simulink model "PV_PEM_direct_battery_active"  (R2026a)
settings: Solver=VariableStepAuto  StopTime=sim_t
values from neighbouring files (symbols this model uses):
  Bi_L = 4e-4    (= 0.0004)    [PV_PEM_direct_battery_active.m]    (also in PV_PEM_direct_battery_passive.m; PV_PEM_indirect_battery.m; PV_PEM_reconfigurable_battery.m)
  Irr_stair_time = (0:Irr_stair_tsamp:sim_t)'    [PV_PEM_direct_battery_active.m]    (also in PV_PEM_direct_battery_passive.m = 0:Irr_stair_tsamp:sim_t; PV_PEM_indirect_battery.m; PV_PEM_reconfigurable_battery.m = (0 : Irr_stair_tsamp : sim_t)')
  Irr_stair_val = interp1(Irr_time, Irr_val, Irr_stair_time, 'linear', 0)    [PV_PEM_direct_battery_active.m]    (also in PV_PEM_direct_battery_passive.m; PV_PEM_indirect_battery.m; PV_PEM_reconfigurable_battery.m = interp1(Irr_time, Irr_val,  Irr_stair_time, 'linear', 0))
  Q_batt = 0.1    [PV_PEM_direct_battery_active.m]    (also in PV_PEM_direct_battery_passive.m; PV_PEM_indirect_battery.m; PV_PEM_reconfigurable_battery.m = 0.00694444444444)
  Ra_stack = Ra   * N    (= 0.02301)    [PV_PEM_direct_battery_active.m]    (also in PV_PEM_direct_battery_passive.m; PV_PEM_indirect_battery.m = 0.0177; PV_PEM_reconfigurable_battery.m = 0.02832)
  Rc_stack = Rc   * N    (= 0.0065)    [PV_PEM_direct_battery_active.m]    (also in PV_PEM_direct_battery_passive.m; PV_PEM_indirect_battery.m = 0.005; PV_PEM_reconfigurable_battery.m = 0.008)
  Rint_stack = Rint * N    (= 0.112749)    [PV_PEM_direct_battery_active.m]    (also in PV_PEM_direct_battery_passive.m; PV_PEM_indirect_battery.m = 0.08673; PV_PEM_reconfigurable_battery.m = 0.138768)
  sample_output_time = 1e-3    (= 0.001)    [PV_PEM_direct_battery_active.m]    (also in PV_PEM_direct_battery_passive.m = 0.0001; PV_PEM_indirect_battery.m = 0.01; PV_PEM_reconfigurable_battery.m = 0.00166666666667)
  SOC_max = 0.9    [PV_PEM_direct_battery_active.m]    (also in PV_PEM_direct_battery_passive.m = 90; PV_PEM_indirect_battery.m; PV_PEM_reconfigurable_battery.m = 90)
  SOC_min = 0.2    [PV_PEM_direct_battery_active.m]    (also in PV_PEM_direct_battery_passive.m = 20; PV_PEM_indirect_battery.m; PV_PEM_reconfigurable_battery.m = 20)
  Ts = 1e-4    (= 0.0001)    [PV_PEM_direct_battery_active.m]    (also in PV_PEM_direct_battery_passive.m; PV_PEM_indirect_battery.m = 0.001; PV_PEM_reconfigurable_battery.m)
  V_ref_battery = (Vint_stack + Vmax_PEM) / 2.1    (= 21.5171109524)    [PV_PEM_direct_battery_active.m]    (also in PV_PEM_direct_battery_passive.m = 22.5929665; PV_PEM_indirect_battery.m = 17.379205; PV_PEM_reconfigurable_battery.m = 27.806728)
libraries: fl_lib x18, nesl_utility x13, simulink x4, ee_lib x3, batteryecm_lib x1, slpidlib x1
settings Model: Creator=hanna  LastModifiedBy=Diamantis
settings SimscapeCC: SimscapeNominalValues="[{\"value\":\"1\",\"unit\":\"A\"},{\"value\":\"1\",\"unit\":\"bar\"},{\"value\":\"1\",\"unit\":\"cm^2\"},{\"value\":\"1\",\"unit\":\"cm^3/s\"},{\"value\":\"1\",\"unit\":\"kJ/kg\"},{\"value\":\"1\",\"unit\":\"kW\"},{\"value\":\"1\",\"unit\":\"l\"},{\"value\":\"1\",\"unit\":\"N\"},{\"value\":\"1\",\"unit\":\"N*m\"},{\"value\":\"1\",\"unit\":\"V\"}]"  SimscapeLogType=none  SimscapeLogDataHistory=5000.0

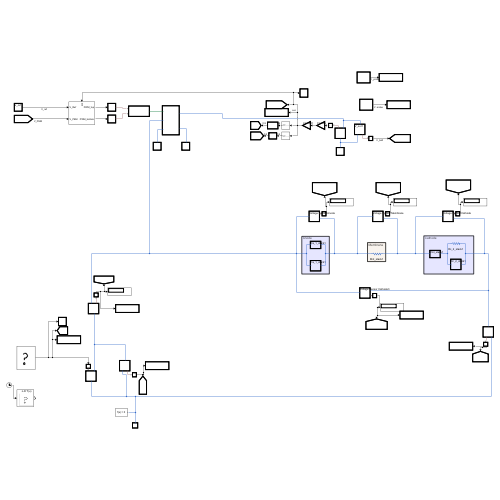
[thumbnail: Simulink's stored preview of the top-level diagram]
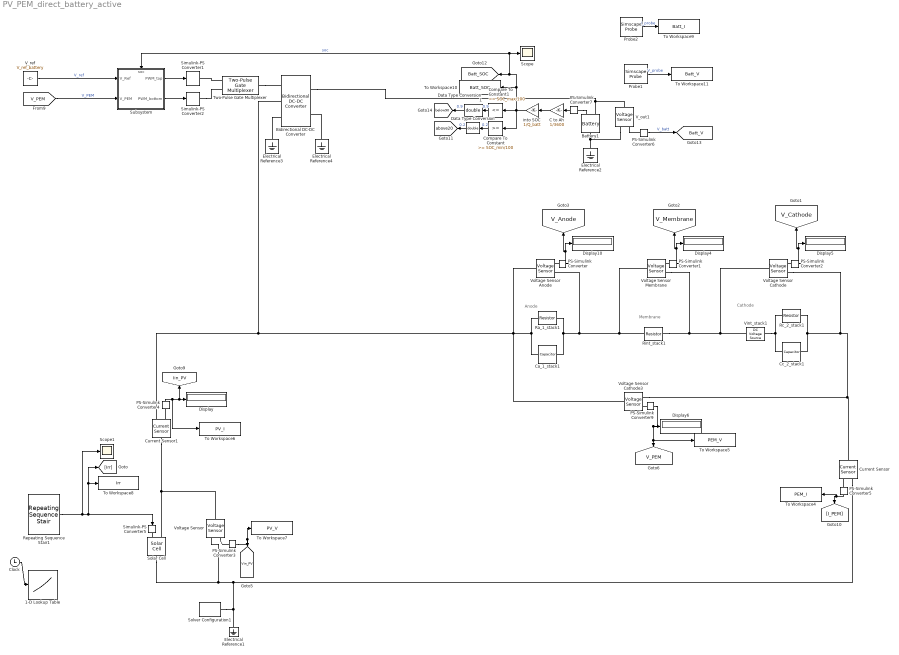
== system PV_PEM_direct_battery_active ==
  note: Membrane
  note: Cathode
  note: Anode
  1-D Lookup Table : Lookup_n-D  NumberOfTableDimensions=1  BreakpointsForDimension1=Irr_stair_time  Table=Irr_stair_val  InternalRulePriority=Speed  RndMeth=Simplest
  Battery1 : batteryecm_lib/Battery  Vnom=V_batt_nom V  prm_dir=simscape.enum.battery.prm_dir.disabled  R1_dis=0.05 Ohm  R1_ch=0.05 Ohm  R1=0.01 Ohm  prm_AH=simscape.enum.battery.prm_AH.finite  AH=Q_batt A*hr  V1=11.5 V  AH1=Q_batt*(SOC_min/100) A*hr  prm_R2=simscape.enum.battery.prm_R2.disabled  R2=2000 Ohm  Tmeas=298.15 K  charge_measurement_port=simscape.enum.battery.enable.yes  prm_dyn=simscape.enum.battery.prm_dyn.off  Rp1=0.005 Ohm  tau1=30 s  Rp2=0.005 Ohm  tau2=30 s  Rp3=0.005 Ohm  tau3=30 s  Rp4=0.005 Ohm  tau4=30 s  Rp5=0.005 Ohm  tau5=30 s  prm_fade=simscape.enum.battery.prm_fade.disabled  N_fade=100  AH_fade=45 A*hr  R1_fade=2.02 Ohm  R1_ch_fade=2.02 Ohm  V1_fade=10.35 V  prm_age=simscape.enum.battery.prm_age.disabled  prm_age_OCV=simscape.enum.battery.prm_age_OCV.OCV  OCV_age=0.9  SOC_age=60  Tmeas_age=298.15 K  delta_time_age_vec=[0] d  temperature_age_vec=[273] K  OCV_scaling_age=2.2134e6  OCV_offset_age=1.632e6  temp_exp_age=0.515833569 V  t_exp_age=0.75  Vnom_T2=12 V  R1_T2=2.2 Ohm  R1_T2_dis=2.2 Ohm  R1_T2_ch=2.2 Ohm  V1_T2=11.4 V  R2_T2=2200 Ohm  Rp1_T2=0.005 Ohm  tau1_T2=30 s  Rp2_T2=0.005 Ohm  tau2_T2=30 s  Rp3_T2=0.005 Ohm  tau3_T2=30 s  Rp4_T2=0.005 Ohm  tau4_T2=30 s  Rp5_T2=0.005 Ohm  tau5_T2=30 s  Tmeas2=273.15 K  thermal_port=simscape.enum.thermaleffects.omit  thermal_mass=30000 J/K  i_specify=off  i_priority=None  i=0 A  i_nominal_specify=off  i_nominal_value=1  i_nominal_unit=A  v_specify=off  v_priority=None  v=0 V  v_nominal_specify=off  v_nominal_value=1  v_nominal_unit=V  charge_specify=on  charge_priority=High  charge=SOC_init A*hr  charge_nominal_specify=off  charge_nominal_value=1  charge_nominal_unit=A*hr  num_cycles_specify=off  num_cycles_priority=High  num_cycles=0  num_cycles_nominal_specify=off  num_cycles_nominal_value=1  num_cycles_nominal_unit=1  temperature_specify=off  temperature_priority=High  temperature=298.15 K  temperature_nominal_specify=off  temperature_nominal_value=1  temperature_nominal_unit=K
      settings: LibrarySourceBlock=batt_lib/Cells/Battery
  Bidirectional DC-DC Converter : ee_lib/Semiconductors & Converters/Converters/Bidirectional DC-DC Converter  fidelity_option=ee.enum.converters.fidelity.detailed  device_type=ee.enum.converters.switchingdevice.mosfet  Vf=0.8 V  Ron=0.001 Ohm  Rds=0.001 Ohm  Goff=1e-6 1/Ohm  Vth=2 V  Vgt=0.5 V  Vgt_off=-1 V  Ih=1 A  K=0  diode_param=ee.enum.converters.diode.nodynamics  diode_Vf=0.8 V  diode_Ron=0.001 Ohm  diode_Goff=1e-5 1/Ohm  diode_C=50 nF  diode_iRM=-5 A  diode_iF=50 A  diode_idot=-50 A/us  diode_trr_param=ee.enum.converters.diodetrr.trr_factor  diode_trr_factor=3  diode_trr=0.5 us  diode_Qrr=1500 s*uA  L=Bi_L H  Rl=0 Ohm  C1=Bi_C1 F  C2=Bi_C2 F  R1=Bi_R1 Ohm  R2=Bi_R2 Ohm  snubber_type=ee.enum.converters.snubber.exclude  Cs=1e-7 F  Rs=0.1 Ohm  iL_specify=off  iL_priority=High  iL=0 A  iL_nominal_specify=off  iL_nominal_value=1  iL_nominal_unit=A  vc1_specify=off  vc1_priority=High  vc1=0 V  vc1_nominal_specify=off  vc1_nominal_value=1  vc1_nominal_unit=V  vc2_specify=off  vc2_priority=High  vc2=0 V  vc2_nominal_specify=off  vc2_nominal_value=1  vc2_nominal_unit=V  device_type_hv=ee.enum.converters.switchingdevice.ideal  Vf_hv=0.8 V  Ron_hv=0.001 Ohm  Rds_hv=0.001 Ohm  Goff_hv=1e-5 1/Ohm  Vth_hv=0.5 V  Vgt_hv=0.5 V  Vgt_off_hv=-1 V  Ih_hv=1 A  device_type_lv=ee.enum.converters.switchingdevice.ideal  Vf_lv=0.8 V  Ron_lv=0.001 Ohm  Rds_lv=0.001 Ohm  Goff_lv=1e-5 1/Ohm  Vth_lv=0.5 V  Vgt_lv=0.5 V  Vgt_off_lv=-1 V  Ih_lv=1 A  T_L1=0.03 H  T_L2=0.03 H  T_k=0.9  snubber_type_hv=ee.enum.converters.snubber.exclude  Cs_hv=1e-7 F  Rs_hv=0.1 Ohm  snubber_type_lv=ee.enum.converters.snubber.exclude  Cs_lv=1e-7 F  Rs_lv=0.1 Ohm  iL1_specify=off  iL1_priority=High  iL1=0 A  iL1_nominal_specify=off  iL1_nominal_value=1  iL1_nominal_unit=A  iL2_specify=off  iL2_priority=High  iL2=0 A  iL2_nominal_specify=off  iL2_nominal_value=1  iL2_nominal_unit=A  hysteresisCurrent=0.01 A
  C to Ah : Gain  Gain=1/3600
  Ca_1_stack1 : fl_lib/Electrical/Electrical Elements/Capacitor  c=Ca_stack F  r=1e-6 Ohm  g=0 1/Ohm  i_specify=off  i_priority=None  i=0 A  i_nominal_specify=off  i_nominal_value=1  i_nominal_unit=A  v_specify=off  v_priority=None  v=0 V  v_nominal_specify=off  v_nominal_value=1  v_nominal_unit=V  vc_specify=off  vc_priority=High  vc=0 V  vc_nominal_specify=off  vc_nominal_value=1  vc_nominal_unit=V
  Cc_2_stack1 : fl_lib/Electrical/Electrical Elements/Capacitor  c=Cc_stack F  r=1e-6 Ohm  g=0 1/Ohm  i_specify=off  i_priority=None  i=0 A  i_nominal_specify=off  i_nominal_value=1  i_nominal_unit=A  v_specify=off  v_priority=None  v=0 V  v_nominal_specify=off  v_nominal_value=1  v_nominal_unit=V  vc_specify=off  vc_priority=High  vc=0 V  vc_nominal_specify=off  vc_nominal_value=1  vc_nominal_unit=V
  Clock : Clock
  Compare To Constant : simulink/Logic and Bit Operations/Compare To Constant  relop=>=  const=SOC_min/100  OutDataTypeStr=boolean
  Compare To Constant1 : simulink/Logic and Bit Operations/Compare To Constant  relop=<=  const=SOC_max/100  OutDataTypeStr=boolean
  Current Sensor : fl_lib/Electrical/Electrical Sensors/Current Sensor
  Current Sensor1 : fl_lib/Electrical/Electrical Sensors/Current Sensor
  Data Type Conversion : DataTypeConversion  OutDataTypeStr=double  SaturateOnIntegerOverflow=off  RndMeth=Floor
  Data Type Conversion1 : DataTypeConversion  OutDataTypeStr=double  SaturateOnIntegerOverflow=off  RndMeth=Floor
  Display{,4..6,10} (5 alike) : Display
  Electrical Reference{1..4} (4 alike) : fl_lib/Electrical/Electrical Elements/Electrical Reference
  PS-Simulink Converter{,1..2,5..7,9} (7 alike) : nesl_utility/PS-Simulink Converter  PhysicalDomain=network_engine_domain  SubClassName=ps_output  LeftPortType=input  RightPortType=output  PseudoPeriodic=off  Frequencies=[]  VectorFormat=inherit  Unit=inherit  AffineConversion=off
  PS-Simulink Converter3 : nesl_utility/PS-Simulink Converter  PhysicalDomain=network_engine_domain  SubClassName=ps_output  LeftPortType=input  RightPortType=output  PseudoPeriodic=off  Frequencies=[]  VectorFormat=1-D array  Unit=V  AffineConversion=off
  PS-Simulink Converter4 : nesl_utility/PS-Simulink Converter  PhysicalDomain=network_engine_domain  SubClassName=ps_output  LeftPortType=input  RightPortType=output  PseudoPeriodic=off  Frequencies=[]  VectorFormat=1-D array  Unit=A  AffineConversion=off
  Probe1 : SimscapeProbe  BoundBlock=499  Variables="{\"i\":{\"Probing\":\"OFF\"},\"n.v\":{\"Probing\":\"OFF\"},\"p.v\":{\"Probing\":\"OFF\"},\"v\":{\"Probing\":\"ON\"}}"
  Probe2 : SimscapeProbe  BoundBlock=499  Variables="{\"i\":{\"Probing\":\"ON\"}}"
  Ra_1_stack1 : fl_lib/Electrical/Electrical Elements/Resistor  R=Ra_stack Ohm  i_specify=off  i_priority=None  i=0 A  i_nominal_specify=off  i_nominal_value=1  i_nominal_unit=A  v_specify=off  v_priority=None  v=0 V  v_nominal_specify=off  v_nominal_value=1  v_nominal_unit=V
  Rc_2_stack1 : fl_lib/Electrical/Electrical Elements/Resistor  R=Rc_stack Ohm  i_specify=off  i_priority=None  i=0 A  i_nominal_specify=off  i_nominal_value=1  i_nominal_unit=A  v_specify=off  v_priority=None  v=0 V  v_nominal_specify=off  v_nominal_value=1  v_nominal_unit=V
  Repeating Sequence Stair1 : simulink/Sources/Repeating Sequence Stair  OutValues=Irr_stair_val  tsamp=Irr_stair_tsamp  OutMin=[]  OutMax=[]  OutDataTypeStr=double  OutputDataTypeScalingMode=double  OutDataType=fixdt(0,8)  ConRadixGroup=Best Precision: Vector-wise  OutScaling=2^-12
  Rint_stack1 : fl_lib/Electrical/Electrical Elements/Resistor  R=Rint_stack Ohm  i_specify=off  i_priority=None  i=0 A  i_nominal_specify=off  i_nominal_value=1  i_nominal_unit=A  v_specify=off  v_priority=None  v=0 V  v_nominal_specify=off  v_nominal_value=1  v_nominal_unit=V
  Scope : Scope
      settings: ActiveDisplayYMinimum=0.599999044089406  ActiveDisplayYMaximum=0.60000010621228816  DataLoggingVariableName=ScopeData4
  Scope1 : Scope
      settings: ActiveDisplayYMinimum=-124.99999999999997  ActiveDisplayYMaximum=1125
  Simulink-PS Converter1 : nesl_utility/Simulink-PS Converter  PhysicalDomain=network_engine_domain  SubClassName=ps_input  LeftPortType=input  RightPortType=output  PseudoPeriodic=off  Frequencies=[]  NoiseDistribution=none  NoiseParameters=[]  Unit=1  AffineConversion=off  FilteringAndDerivatives=provide  SimscapeFilterOrder=1  InputFilterTimeConstant=1e-7  UdotUserProvided=0
  Simulink-PS Converter2 : nesl_utility/Simulink-PS Converter  PhysicalDomain=network_engine_domain  SubClassName=ps_input  LeftPortType=input  RightPortType=output  PseudoPeriodic=off  Frequencies=[]  NoiseDistribution=none  NoiseParameters=[]  Unit=1  AffineConversion=off  FilteringAndDerivatives=provide  SimscapeFilterOrder=1  InputFilterTimeConstant=1e-7  UdotUserProvided=0
  Simulink-PS Converter5 : nesl_utility/Simulink-PS Converter  PhysicalDomain=network_engine_domain  SubClassName=ps_input  LeftPortType=input  RightPortType=output  PseudoPeriodic=off  Frequencies=[]  NoiseDistribution=none  NoiseParameters=[]  Unit=1  AffineConversion=off  FilteringAndDerivatives=provide  SimscapeFilterOrder=1  InputFilterTimeConstant=0.001  UdotUserProvided=0
  Solar Cell : ee_lib/Sources/Solar Cell  PartSpecification="{\"CollectionId\":\"SimscapeElectrical\",\"CollectionVersion\":\"1.0.0\",\"DatasetId\":\"Amerisolar|AS_6M30_HC_320W|simscape.electrical.solarCell\",\"DisplayName\":\"Amerisolar:AS_6M30_HC_320W\"}"  prm=3  Isc=10.14 % Datasheet derived A  Voc=0.67 % Datasheet derived V  Is=3.24823447983853e-07 % Datasheet derived A  Is2=9.37081970792037e-10 % Datasheet derived A  Iph=10.140005507508 % Datasheet derived A  Ir0=1000 % Datasheet derived W/m^2  ec=1.51118472243322 % Datasheet derived  N2=2.60259908345858 % Datasheet derived  Rs=1.94548269975201e-05 % Datasheet derived Ohm  Rp=682.95993142779 % Datasheet derived Ohm  N_series=Ns_cell % Datasheet derived  N_parallel=Np_cell % Datasheet derived  TIPH1=0.000499942933005141 % Datasheet derived 1/K  EG=1.12 % Datasheet derived eV  TXIS1=4.23641510120988 % Datasheet derived  TXIS2=16.2689137700667 % Datasheet derived  TRS1=0.243341028305912 % Datasheet derived  TRP1=0 % Parameter not set  Tmeas=25 % Datasheet derived degC  TFIXED=25 % Datasheet derived degC  thermal_mass=100 % Parameter not set J/K  initial_temperature=25 degC
      settings: AttributesFormatString=Amerisolar:AS_6M30_HC_320W
  Solver Configuration1 : nesl_utility/Solver Configuration  PhysicalDomain=network_engine_domain  SubClassName=solver  LeftPortType=input  RightPortType=generic  Tones=[]  Harmonics=[]  SimulateNoise=off  Profile=off  UseLocalSampling=off  EnableSwitchedLinearOptims=on  FrequencyDomain=off  UseCCode=off  RelTol=0.001  AbsTol=0.001  MinStep=1e-09  ToWorkspace=off  RevertToSquareIcSolve=off  NumHomotopyIterations=100  PhasorMode=off  PhasorModeNumHarmonics=1  ConsistencySolver=NEWTON_XTOL_AFTER_FTOL  CanonicalOrdering=UNORDERED  OptimizeIntermediates=UNOPTIMIZED  IndexReductionMethod=DerivativeReplacement  DoDC=off  ResidualTolerance=1e-09  ConsistencyTolSource=GLOBAL  ConsistencyAbsTol=0.001  ConsistencyRelTol=0.001  ConsistencyTolFactor=0.001  UseLocalSolver=off  LocalSolverChoice=NE_BACKWARD_EULER_ADVANCER  ResolveIndetEquations=on  FunctionEvalNumThread=1  LocalSolverSampleTime=0.001  DoFixedCost=off  MaxNonlinIter=3  MaxModeIter=2  ComputeImpulses=off  ImpulseIterations=2  LinearAlgebra=auto  LinearAlgebraNumThread=0  EquationFormulation=NE_TIME_EF  DelaysMemoryBudget=1024  AutomaticFiltering=on  FilteringTimeConstant=0.001  PartitionStorageMethod=AS_NEEDED  PartitionMemoryBudget=1024  PartitionMethod=ROBUST  MultibodyUseLocalSolver=off  MultibodyLocalSolverChoice=ODE1  MultibodyLocalSolverSampleTime=0.001
  Subsystem : Subsystem
      settings: PortSchema="{\"entries\":[{\"content\":{\"sides\":[{\"content\":{\"connectorIds\":[\"In1\",\"In2\"]},\"type\":\"ConnectorPlacement.EquallySpacedRectSide\",\"uuid\":\"4e9ec41c-bdf9-454a-9c62-b3d400a7e8a5\"},{\"content\":{\"connectorIds\":[\"Out1\",\"Out2\"],\"side\":\"RIGHT\"},\"type\":\"ConnectorPlacement.EquallySpacedRectSide\",\"uuid\":\"9c7ad0fb-9491-4539-a93e-b9f6c9148e2a\"},{\"content\":{\"connectorIds\":[\"In3\"],\"side\":\"TOP\"},\"type\":\"ConnectorPlacement.EquallySpacedRectSide\",\"uuid\":\"b08aae61-0a78-4c70-83b8-04326ad74e93\"}]},\"type\":\"ConnectorPlacement.EquallySpacedConnector\",\"uuid\":\"604710b3-7757-4fb6-916a-2f806a8ce5d4\"}],\"packageUris\":[\"http://schema.mathworks.com/mf0/Connector/R2020b\"],\"version\":\"1.0\"}"
  To Workspace10 : ToWorkspace  VariableName=Batt_SOC  SaveFormat=Timeseries  SampleTime=sample_output_time
  To Workspace11 : ToWorkspace  VariableName=Batt_V  SaveFormat=Timeseries  SampleTime=sample_output_time
  To Workspace4 : ToWorkspace  VariableName=PEM_I  SaveFormat=Timeseries  SampleTime=sample_output_time
  To Workspace5 : ToWorkspace  VariableName=PEM_V  SaveFormat=Timeseries  SampleTime=sample_output_time
  To Workspace6 : ToWorkspace  VariableName=PV_I  SaveFormat=Timeseries  SampleTime=sample_output_time
  To Workspace7 : ToWorkspace  VariableName=PV_V  SaveFormat=Timeseries  SampleTime=sample_output_time
  To Workspace8 : ToWorkspace  VariableName=Irr  SaveFormat=Timeseries  SampleTime=sample_output_time
  To Workspace9 : ToWorkspace  VariableName=Batt_I  SaveFormat=Timeseries  SampleTime=sample_output_time
  Two-Pulse Gate Multiplexer : ee_lib/Semiconductors & Converters/Converters/Two-Pulse Gate Multiplexer  port_option=ee.enum.controlport.ps
  V_out1 : fl_lib/Electrical/Electrical Sensors/Voltage Sensor
  V_ref : Constant  Value=V_ref_battery
  Vint_stack1 : fl_lib/Electrical/Electrical Sources/DC Voltage Source  v0=Vint_stack V
  Voltage Sensor : fl_lib/Electrical/Electrical Sensors/Voltage Sensor
  Voltage Sensor Anode : fl_lib/Electrical/Electrical Sensors/Voltage Sensor
  Voltage Sensor Cathode : fl_lib/Electrical/Electrical Sensors/Voltage Sensor
  Voltage Sensor Cathode3 : fl_lib/Electrical/Electrical Sensors/Voltage Sensor
  Voltage Sensor Membrane : fl_lib/Electrical/Electrical Sensors/Voltage Sensor
  into SOC : Gain  Gain=1/Q_batt
  tag scope: Batt_SOC=global, Batt_V=global, Iin_PV=global, V_Anode=global, V_Cathode=global, V_Membrane=global, V_PEM=global, Vin_PV=global, above20=global, below90=global
  wires:
  Repeating Sequence Stair1/1 -> Simulink-PS Converter5/1, To Workspace8/1, [Irr], Scope1/1
  Clock/1 -> 1-D Lookup Table/1
  PS-Simulink Converter1/1 -> [V_Membrane], Display4/1
  PS-Simulink Converter9/1 -> To Workspace5/1, [V_PEM], Display6/1
  PS-Simulink Converter/1 -> [V_Anode], Display10/1
  PS-Simulink Converter2/1 -> [V_Cathode], Display5/1
  PS-Simulink Converter4/1 -> To Workspace6/1, [Iin_PV], Display/1
  PS-Simulink Converter5/1 -> To Workspace4/1, [I_PEM]
  PS-Simulink Converter3/1 -> To Workspace7/1, [Vin_PV]
  Compare To Constant1/1 -> Data Type Conversion1/1  "0.9"
  Compare To Constant/1 -> Data Type Conversion/1  "0.2"
  into SOC/1 -> Compare To Constant1/1, To Workspace10/1, [Batt_SOC], Subsystem/3(soc), Scope/1, Compare To Constant/1  "soc"
  Data Type Conversion1/1 -> [below90]  "0.9"
  Subsystem/1(PWM_top) -> Simulink-PS Converter1/1
  C to Ah/1 -> into SOC/1
  Probe1/1 -> To Workspace11/1  "V_probe"
  PS-Simulink Converter7/1 -> C to Ah/1
  Subsystem/2(PWM_bottom) -> Simulink-PS Converter2/1
  [V_PEM] -> Subsystem/2(V_PEM)  "V_PEM"
  PS-Simulink Converter6/1 -> [Batt_V]  "V_batt"
  Data Type Conversion/1 -> [above20]  "0.2"
  Probe2/1 -> To Workspace9/1  "I_probe"
  V_ref/1 -> Subsystem/1(V_Ref)  "V_ref"
  connections:
  Solver Configuration1/RConn1 -- Voltage Sensor/RConn2 -- Solar Cell/RConn1 -- Current Sensor/RConn2 -- Electrical Reference1/LConn1
  Simulink-PS Converter5/RConn1 -- Solar Cell/LConn1
  Current Sensor1/LConn1 -- Voltage Sensor/LConn1 -- Solar Cell/LConn2
  Voltage Sensor Anode/RConn2 -- Ra_1_stack1/RConn1 -- Ca_1_stack1/RConn1 -- Rint_stack1/LConn1 -- Voltage Sensor Membrane/LConn1
  Voltage Sensor Anode/LConn1 -- Current Sensor1/RConn2 -- Bidirectional DC-DC Converter/LConn2 -- Voltage Sensor Cathode3/LConn1 -- Ca_1_stack1/LConn1 -- Ra_1_stack1/LConn1
  Voltage Sensor Membrane/RConn2 -- Voltage Sensor Cathode/LConn1 -- Vint_stack1/LConn1 -- Rint_stack1/RConn1
  Cc_2_stack1/RConn1 -- Rc_2_stack1/RConn1 -- Current Sensor/LConn1 -- Voltage Sensor Cathode3/RConn2 -- Voltage Sensor Cathode/RConn2
  Cc_2_stack1/LConn1 -- Vint_stack1/RConn1 -- Rc_2_stack1/LConn1
  Voltage Sensor Cathode3/RConn1 -- PS-Simulink Converter9/LConn1
  Voltage Sensor Membrane/RConn1 -- PS-Simulink Converter1/LConn1
  Voltage Sensor Cathode/RConn1 -- PS-Simulink Converter2/LConn1
  Voltage Sensor Anode/RConn1 -- PS-Simulink Converter/LConn1
  Current Sensor1/RConn1 -- PS-Simulink Converter4/LConn1
  PS-Simulink Converter5/LConn1 -- Current Sensor/RConn1
  PS-Simulink Converter3/LConn1 -- Voltage Sensor/RConn1
  Bidirectional DC-DC Converter/RConn1 -- V_out1/LConn1 -- Battery1/LConn1
  Battery1/RConn1 -- V_out1/RConn2 -- Electrical Reference2/LConn1
  Electrical Reference3/LConn1 -- Bidirectional DC-DC Converter/LConn3
  Two-Pulse Gate Multiplexer/RConn1 -- Bidirectional DC-DC Converter/LConn1
  V_out1/RConn1 -- PS-Simulink Converter6/LConn1
  PS-Simulink Converter7/LConn1 -- Battery1/LConn2
  Electrical Reference4/LConn1 -- Bidirectional DC-DC Converter/RConn2
  Simulink-PS Converter2/RConn1 -- Two-Pulse Gate Multiplexer/LConn2
  Two-Pulse Gate Multiplexer/LConn1 -- Simulink-PS Converter1/RConn1

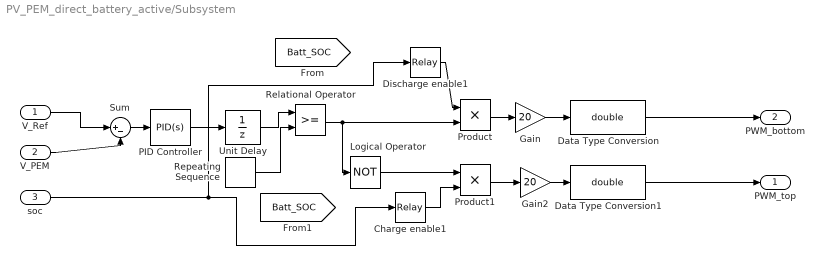
== system PV_PEM_direct_battery_active/Subsystem ==
  V_Ref : Inport
  V_PEM : Inport  Port=2
  soc : Inport  Port=3
  Charge enable1 : Relay  OnSwitchValue=0.9  OffSwitchValue=0.85  OnOutputValue=0  OffOutputValue=1
  Data Type Conversion : DataTypeConversion  OutDataTypeStr=double  SaturateOnIntegerOverflow=off  RndMeth=Floor
  Data Type Conversion1 : DataTypeConversion  OutDataTypeStr=double  SaturateOnIntegerOverflow=off  RndMeth=Floor
  Discharge enable1 : Relay  OnSwitchValue=0.25  OffSwitchValue=0.2
  Gain : Gain  Gain=20
  Gain2 : Gain  Gain=20
  Logical Operator : Logic  Operator=NOT  AllPortsSameDT=off  OutDataTypeStr=boolean
  PID Controller : slpidlib/PID Controller  Controller=PID  Form=Parallel  TimeDomain=Continuous-time  UseExternalTs=off  SampleTime=-1  IntegratorMethod=Forward Euler  FilterMethod=Forward Euler  ControllerParametersSource=internal  P=0.05  I=15  UseKiTs=off  D=0  UseExternalDerivativeSource=off  N=100  UseFilter=on  TunerSelectOption=Transfer Function Based (PID Tuner App)  InitialConditionSource=internal  InitialConditionForIntegrator=0  InitialConditionForFilter=0  DifferentiatorICPrevScaledInput=0  ExternalReset=none  TrackingMode=off  Kt=1  LimitOutput=off  SatLimitsSource=internal  UpperSaturationLimit=0.9  LowerSaturationLimit=0.1  LinearizeAsGain=on  AntiWindupMode=none  Kb=1  LimitIntegrator=off  UpperIntegratorSaturationLimit=inf  LowerIntegratorSaturationLimit=-inf  POutMin=[]  POutMax=[]  IOutMin=[]  IOutMax=[]  DOutMin=[]  DOutMax=[]  NOutMin=[]  NOutMax=[]  SumOutMin=[]  SumOutMax=[]  SaturationOutMin=[]  SaturationOutMax=[]  PParamMin=[]  PParamMax=[]  IParamMin=[]  IParamMax=[]  DParamMin=[]  DParamMax=[]  NParamMin=[]  NParamMax=[]  KbParamMin=[]  KbParamMax=[]  KtParamMin=[]  KtParamMax=[]  KbOutMin=[]  KbOutMax=[]  KtOutMin=[]  KtOutMax=[]  IntegratorOutMin=[]  IntegratorOutMax=[]  FilterOutMin=[]  FilterOutMax=[]  SumI1OutMin=[]  SumI1OutMax=[]  SumI2OutMin=[]  SumI2OutMax=[]  SumI3OutMin=[]  SumI3OutMax=[]  SumI4OutMin=[]  SumI4OutMax=[]  SumDOutMin=[]  SumDOutMax=[]  DifferentiatorOutMin=[]  DifferentiatorOutMax=[]  FilterDiffOutCoefMin=[]  FilterDiffOutCoefMax=[]  ReciprocalOutMin=[]  ReciprocalOutMax=[]  SumDenOutMin=[]  SumDenOutMax=[]  SumNumOutMin=[]  SumNumOutMax=[]  DivideOutMin=[]  DivideOutMax=[]  UdiffTsProdOutMin=[]  UdiffTsProdOutMax=[]  NTsProdOutMin=[]  NTsProdOutMax=[]  UintegralTsProdOutMin=[]  UintegralTsProdOutMax=[]  UngainTsProdOutMin=[]  UngainTsProdOutMax=[]  ClampingZeroOutDataTypeStr=Inherit: Inherit via back propagation  ClampingZeroOutMin=[]  ClampingZeroOutMax=[]  FilterDenConstantOutDataTypeStr=Inherit: Inherit via back propagation  FilterDenConstantOutMin=[]  FilterDenConstantOutMax=[]  PCopyOutDataTypeStr=Inherit: Inherit via back propagation  PCopyOutMin=[]  PCopyOutMax=[]  NCopyOutDataTypeStr=Inherit: Inherit via back propagation  NCopyOutMin=[]  NCopyOutMax=[]  IntegratorContinuousStateAttributes=''  IntegratorStateMustResolveToSignalObject=off  IntegratorRTWStateStorageClass=Auto  FilterContinuousStateAttributes=''  FilterStateMustResolveToSignalObject=off  FilterRTWStateStorageClass=Auto  ParallelPVariant=InternalParameters  IdealPVariant=Disabled  IVariant=InternalParameters  DVariant=InternalParameters  IntegratorVariant=Continuous  SatVariant=Disabled  AWVariant=Passthrough  PCopyVariant=Disabled  TRVariant=Disabled  FdbkBlocksVariant=Forward  IdealPFdbkVariant=Disabled  SatFdbkVariant=Disabled  DerivativeFilterVariant=ContFilter  NVariant=InternalParameters  NCopyVariant=Disabled  FilterICVariant=InternalICsFilter  IntegratorICVariant=InternalICs  ExternalResetVariant=Disabled  TRSumVariant=Passthrough  SumFdbkVariant=Disabled  SumVariant=Sum_PID  TsampFilterVariant=InternalTs  TsampNgainVariant=Passthrough  TsampIntegralVariant=Disabled_SignalSpec  ExternalSaturationOutDataTypeStr=Inherit: Same as second input  DerivativeSourceVariant=ErrorSignal  PreIntVariant=InternalPreInt
  Product : Product
  Product1 : Product
  Relational Operator : RelationalOperator  OutDataTypeStr=boolean  RndMeth=Simplest  InputSameDT=off
  Repeating Sequence : simulink/Sources/Repeating Sequence  rep_seq_t=[0, 1e-4]  rep_seq_y=[0, 1]
  Sum : Sum  Inputs=|+-
  Unit Delay : UnitDelay  SampleTime=Ts
  PWM_top : Outport  VectorParamsAs1DForOutWhenUnconnected=off
  PWM_bottom : Outport  Port=2  VectorParamsAs1DForOutWhenUnconnected=off
  wires:
  Repeating Sequence/1 -> Relational Operator/2
  Gain/1 -> Data Type Conversion/1
  Gain2/1 -> Data Type Conversion1/1
  PID Controller/1 -> Unit Delay/1
  Relational Operator/1 -> Logical Operator/1, Product/2
  Logical Operator/1 -> Product1/1
  Sum/1 -> PID Controller/1
  V_Ref/1 -> Sum/1
  Unit Delay/1 -> Relational Operator/1
  V_PEM/1 -> Sum/2
  Data Type Conversion/1 -> PWM_bottom/1
  Data Type Conversion1/1 -> PWM_top/1
  Discharge enable1/1 -> Product/1
  Charge enable1/1 -> Product1/2
  Product1/1 -> Gain2/1
  Product/1 -> Gain/1
  soc/1 -> Charge enable1/1, Discharge enable1/1
